simulink model "forceControl"  (R2024b)
settings: Solver=VariableStepAuto  StartTime=0.0  StopTime=10
values from neighbouring files (symbols this model uses):
  robotStructure = block.DialogPrm(1).Data    [activeCompliance.m]    (also in robot.mat = )
undefined symbols (not defined in the file or in its folder): X, Y, Z
libraries: sm_lib x141, nesl_utility x12, matrix_library x3
(part 1 of 3)
settings Model: PacingRate=10000  Creator=luca  LastModifiedBy=luca
settings DebuggingCC: AlgebraicLoopMsg=none

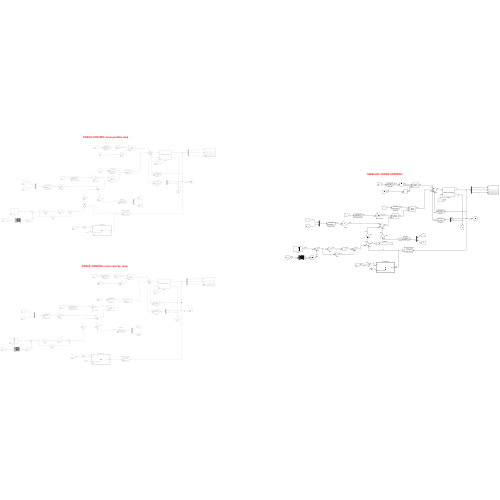
[thumbnail: Simulink's stored preview of the top-level diagram]
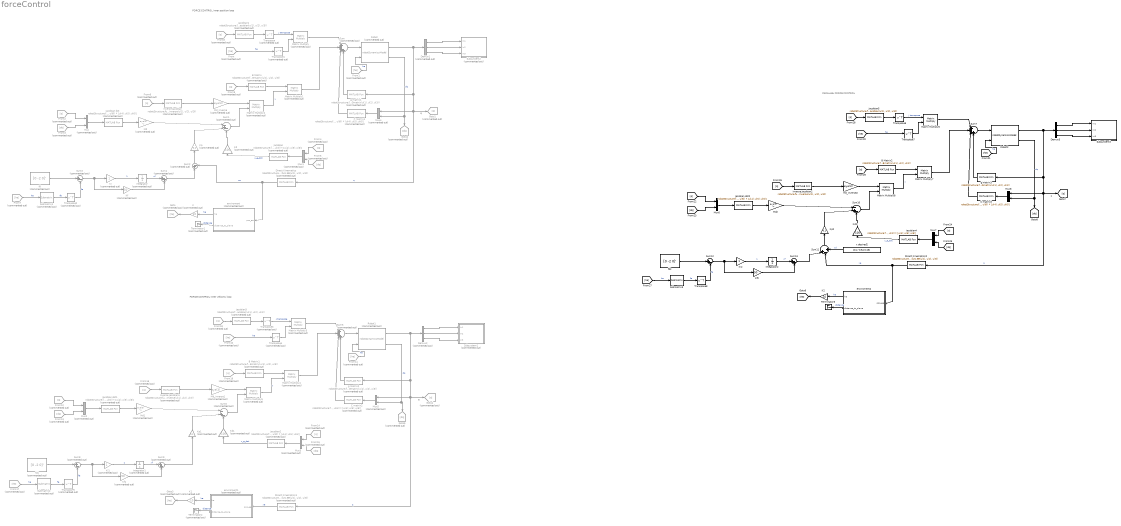
== system forceControl ==
  note: q
  note: FORCE CONTROL inner position loop
  note: q
  note: FORCE CONTROL inner velocity loop
  note: q
  note: PARALLEL FORCE CONTROL
  B Matrix : MATLABFcn  Commented=on  MATLABFcn=robotStructure.func.Bmatrix(u(1), u(2), u(3))  Output1D=off
  B Matrix1 : MATLABFcn  Commented=on  MATLABFcn=robotStructure.func.Bmatrix(u(1), u(2), u(3))  Output1D=off
  B Matrix2 : MATLABFcn  MATLABFcn=robotStructure.func.Bmatrix(u(1), u(2), u(3))  Output1D=off
  C matrix1 : MATLABFcn  Commented=on  MATLABFcn=robotStructure.func.Cmatrix(u(1), u(2), u(3), u(4), u(5), u(6)) * [u(4); u(5); u(6)]  OutputSignalType=real  Output1D=off
  C matrix2 : MATLABFcn  Commented=on  MATLABFcn=robotStructure.func.Cmatrix(u(1), u(2), u(3), u(4), u(5), u(6)) * [u(4); u(5); u(6)]  OutputSignalType=real  Output1D=off
  C matrix3 : MATLABFcn  MATLABFcn=robotStructure.func.Cmatrix(u(1), u(2), u(3), u(4), u(5), u(6)) * [u(4); u(5); u(6)]  OutputSignalType=real  Output1D=off
  Demux1 : Demux  Commented=on  Outputs=3
  Demux2 : Demux  Commented=on  Outputs=3
  Demux3 : Demux  Outputs=3
  Direct Kinematics : MATLABFcn  Commented=on  MATLABFcn=robotStructure.func.EE(u(1), u(2), u(3))  Output1D=off
  Direct Kinematics1 : MATLABFcn  Commented=on  MATLABFcn=robotStructure.func.EE(u(1), u(2), u(3))  Output1D=off
  Direct Kinematics2 : MATLABFcn  MATLABFcn=robotStructure.func.EE(u(1), u(2), u(3))  Output1D=off
  From{,1,7,10..11,17} (6 alike) : From  Commented=on  GotoTag=he
  From{2,4,6,8..9,12,14,16,18..19} (10 alike) : From  Commented=on  GotoTag=q
  From{3,5,13,15} (4 alike) : From  Commented=on  GotoTag=dq
  Goto : Goto  Commented=on  GotoTag=he
  Goto1 : Goto  Commented=on  GotoTag=q
  Goto2 : Goto  Commented=on  GotoTag=dq
  Goto3 : Goto  Commented=on  GotoTag=he
  Goto4 : Goto  Commented=on  GotoTag=q
  Goto5 : Goto  Commented=on  GotoTag=dq
  Integrator : Integrator  Commented=on
  Integrator1 : Integrator  Commented=on
  Integrator2 : Integrator
  K : Gain  Commented=on  Gain=10
  K1 : Gain  Commented=on  Gain=10
  K2 : Gain  Gain=10
  Kd : Gain  Commented=on  Gain=100
  Kd1 : Gain  Commented=on  Gain=100
  Kd2 : Gain  Gain=100
  Kf : Gain  Commented=on  Gain=50
  Kf1 : Gain  Commented=on  Gain=50
  Kf2 : Gain  Gain=50
  Ki : Gain  Commented=on
  Ki1 : Gain  Commented=on
  Ki2 : Gain
  Kp : Gain  Commented=on  Gain=0.1
  Kp1 : Gain  Commented=on  Gain=0.1
  Kp2 : Gain  Gain=0.1
  Matrix Multiply{,1..5} (6 alike) : Product  Commented=on  Multiplication=Matrix(*)
  Matrix Multiply6 : Product  Multiplication=Matrix(*)
  Matrix Multiply7 : Product  Multiplication=Matrix(*)
  Matrix Multiply8 : Product  Multiplication=Matrix(*)
  Md : Gain  Commented=on  Gain=eye(3)  Multiplication=Matrix(K*u)
  Md1 : Gain  Commented=on  Gain=eye(3)  Multiplication=Matrix(K*u)
  Md2 : Gain  Gain=eye(3)  Multiplication=Matrix(K*u)
  Md_inverse : Gain  Commented=on  Gain=eye(3)
  Md_inverse1 : Gain  Commented=on  Gain=eye(3)
  Md_inverse2 : Gain  Gain=eye(3)
  Mux{,1..5} (6 alike) : Mux  Commented=on  Inputs=2
  Mux6 : Mux  Inputs=2
  Mux7 : Mux  Inputs=2
  Mux8 : Mux  Inputs=2
  Robot : M-S-Function  Commented=on  FunctionName=robotDynamicsModel  Parameters=robotStructure, [0 -0.05 0], [0 0 0]
  Robot1 : M-S-Function  Commented=on  FunctionName=robotDynamicsModel  Parameters=robotStructure, [0 -0.05 0], [0 0 0]
  Robot2 : M-S-Function  FunctionName=robotDynamicsModel  Parameters=robotStructure, [0 -0.2 0], [0 0 0]
  Submatrix1 : matrix_library/Submatrix  Commented=on  RowSpan=All rows  RowStartMode=Index  RowStartIndex=1  RowEndMode=Index  RowEndIndex=1  ColSpan=Range of columns  ColStartMode=Index  ColStartIndex=1  ColEndMode=Index  ColEndIndex=3
  Submatrix2 : matrix_library/Submatrix  Commented=on  RowSpan=All rows  RowStartMode=Index  RowStartIndex=1  RowEndMode=Index  RowEndIndex=1  ColSpan=Range of columns  ColStartMode=Index  ColStartIndex=1  ColEndMode=Index  ColEndIndex=3
  Submatrix3 : matrix_library/Submatrix  RowSpan=All rows  RowStartMode=Index  RowStartIndex=1  RowEndMode=Index  RowEndIndex=1  ColSpan=Range of columns  ColStartMode=Index  ColStartIndex=1  ColEndMode=Index  ColEndIndex=3
  Subsystem1 : Subsystem  Commented=on
  Subsystem2 : Subsystem  Commented=on
  Subsystem3 : Subsystem
  Sum : Sum  Commented=on  Inputs=|++++
  Sum1 : Sum  Commented=on  Inputs=|-+-
  Sum10 : Sum  Inputs=|-+-
  Sum11 : Sum  Inputs=|+|-|+
  Sum12 : Sum  Inputs=|+-
  Sum13 : Sum  Inputs=|++
  Sum2 : Sum  Commented=on  Inputs=|+-
  Sum3 : Sum  Commented=on  Inputs=|+-
  Sum4 : Sum  Commented=on  Inputs=|++
  Sum5 : Sum  Commented=on  Inputs=|++++
  Sum6 : Sum  Commented=on  Inputs=|-+-
  Sum7 : Sum  Inputs=|++++
  Sum8 : Sum  Commented=on  Inputs=|+-
  Sum9 : Sum  Commented=on  Inputs=|++
  Terminator1 : Terminator  Commented=on
  Terminator2 : Terminator  Commented=on
  Terminator3 : Terminator
  Transpose{,1..5} (6 alike) : Math  Commented=on  Operator=transpose
  Transpose6 : Math  Operator=transpose
  Transpose7 : Math  Operator=transpose
  Transpose8 : Math  Operator=transpose
  enviroment : MATLAB Function  Commented=on  TreatAsAtomicUnit=on
  enviroment1 : MATLAB Function  Commented=on  TreatAsAtomicUnit=on
  enviroment2 : MATLAB Function  TreatAsAtomicUnit=on
  fd : Constant  Commented=on  Value=[0 -2 0]'  VectorParams1D=off
  fd1 : Constant  Commented=on  Value=[0 -2 0]'  VectorParams1D=off
  fd2 : Constant  Value=[0 -2 0]'  VectorParams1D=off
  g matrix1 : MATLABFcn  Commented=on  MATLABFcn=robotStructure.func.Gmatrix(u(1), u(2), u(3))  OutputSignalType=real  Output1D=off
  g matrix2 : MATLABFcn  Commented=on  MATLABFcn=robotStructure.func.Gmatrix(u(1), u(2), u(3))  OutputSignalType=real  Output1D=off
  g matrix3 : MATLABFcn  MATLABFcn=robotStructure.func.Gmatrix(u(1), u(2), u(3))  OutputSignalType=real  Output1D=off
  inverse Jacobian : MATLABFcn  Commented=on  MATLABFcn=robotStructure.func.AnalitycalJacobianInverse(u(1), u(2), u(3))  Output1D=off
  inverse Jacobian1 : MATLABFcn  Commented=on  MATLABFcn=robotStructure.func.AnalitycalJacobianInverse(u(1), u(2), u(3))  Output1D=off
  inverse Jacobian2 : MATLABFcn  MATLABFcn=robotStructure.func.AnalitycalJacobianInverse(u(1), u(2), u(3))  Output1D=off
  jacobian : MATLABFcn  Commented=on  MATLABFcn=robotStructure.func.AnalitycalJacobian(u(1), u(2), u(3)) * [u(4); u(5); u(6)]  Output1D=off
  jacobian dot : MATLABFcn  Commented=on  MATLABFcn=robotStructure.func.AnalitycalJacobianDot(u(1), u(2), u(3), u(4), u(5), u(6)) * [u(4); u(5); u(6)]  Output1D=off
  jacobian dot1 : MATLABFcn  Commented=on  MATLABFcn=robotStructure.func.AnalitycalJacobianDot(u(1), u(2), u(3), u(4), u(5), u(6)) * [u(4); u(5); u(6)]  Output1D=off
  jacobian dot2 : MATLABFcn  MATLABFcn=robotStructure.func.AnalitycalJacobianDot(u(1), u(2), u(3), u(4), u(5), u(6)) * [u(4); u(5); u(6)]  Output1D=off
  jacobian1 : MATLABFcn  Commented=on  MATLABFcn=robotStructure.func.GeometricJacobian(u(1), u(2), u(3))  Output1D=off
  jacobian2 : MATLABFcn  Commented=on  MATLABFcn=robotStructure.func.AnalitycalJacobian(u(1), u(2), u(3)) * [u(4); u(5); u(6)]  Output1D=off
  jacobian3 : MATLABFcn  Commented=on  MATLABFcn=robotStructure.func.GeometricJacobian(u(1), u(2), u(3))  Output1D=off
  jacobian4 : MATLABFcn  MATLABFcn=robotStructure.func.AnalitycalJacobian(u(1), u(2), u(3)) * [u(4); u(5); u(6)]  Output1D=off
  jacobian5 : MATLABFcn  MATLABFcn=robotStructure.func.GeometricJacobian(u(1), u(2), u(3))  Output1D=off
  x desired2 : Constant  Value=[0.4 -0.54 0.15]
  wires:
  enviroment/2(distance_to_plane) -> Terminator1/1  "distance"
  Demux1/2 -> Subsystem2/2(In2)
  Robot/1 -> g matrix1/1, Goto1/1, Mux4/1, Direct Kinematics/1, Demux1/1  "q"
  Demux1/1 -> Subsystem2/1(In1)
  Demux1/3 -> Subsystem2/3(In3)
  Sum/1 -> Robot/1
  Robot/2 -> Mux4/2, Goto2/1  "dq"
  Mux4/1 -> C matrix1/1
  enviroment/1(he) -> K/1  "he"
  g matrix1/1 -> Sum/4
  C matrix1/1 -> Sum/3
  From1/1 -> Robot/2  "he"
  Direct Kinematics/1 -> Sum2/2, enviroment/1(pos_ee)  "xe"
  B Matrix/1 -> Matrix Multiply1/1
  Matrix Multiply2/1 -> Matrix Multiply1/2  "y"
  inverse Jacobian/1 -> Md_inverse/1
  Md_inverse/1 -> Matrix Multiply2/1
  Sum1/1 -> Matrix Multiply2/2
  Kd/1 -> Sum1/3
  jacobian/1 -> Kd/1  "x_e_dot"
  Kp/1 -> Sum1/2
  Sum2/1 -> Kp/1
  jacobian dot/1 -> Md/1
  Md/1 -> Sum1/1
  From2/1 -> Mux/1
  Mux/1 -> jacobian dot/1
  From3/1 -> Mux/2
  From/1 -> Transpose1/1  "he"
  From5/1 -> Mux1/2
  From4/1 -> Mux1/1
  Mux1/1 -> jacobian/1
  From6/1 -> inverse Jacobian/1
  From9/1 -> B Matrix/1
  Transpose2/1 -> Sum3/2  "fe"
  Submatrix1/1 -> Transpose2/1  "fe"
  From7/1 -> Submatrix1/1  "he"
  fd/1 -> Sum3/1
  Sum3/1 -> Kf/1, Ki/1
  Ki/1 -> Integrator/1  "1"
  Integrator/1 -> Sum4/1  "xf"
  Sum4/1 -> Sum2/1
  K/1 -> Goto/1
  Matrix Multiply1/1 -> Sum/2
  Matrix Multiply/1 -> Sum/1
  From8/1 -> jacobian1/1
  jacobian1/1 -> Transpose/1
  Transpose/1 -> Matrix Multiply/1  "J transpose"
  Transpose1/1 -> Matrix Multiply/2
  Kf/1 -> Sum4/2
  Sum8/1 -> Kf1/1, Ki1/1
  Kf1/1 -> Sum9/2
  From17/1 -> Submatrix2/1  "he"
  Md1/1 -> Sum6/1
  inverse Jacobian1/1 -> Md_inverse1/1
  g matrix2/1 -> Sum5/4
  Ki1/1 -> Integrator1/1  "1"
  Mux5/1 -> C matrix2/1
  C matrix2/1 -> Sum5/3
  Robot1/1 -> g matrix2/1, Goto4/1, Mux5/1, Direct Kinematics1/1, Demux2/1  "q"
  enviroment1/2(distance_to_plane) -> Terminator2/1  "distance"
  From19/1 -> B Matrix1/1
  From16/1 -> inverse Jacobian1/1
  From13/1 -> Mux2/2
  Direct Kinematics1/1 -> enviroment1/1(pos_ee)  "xe"
  Sum6/1 -> Matrix Multiply5/2
  Matrix Multiply3/1 -> Sum5/1
  Sum5/1 -> Robot1/1
  B Matrix1/1 -> Matrix Multiply4/1
  From11/1 -> Robot1/2  "he"
  Transpose4/1 -> Matrix Multiply3/2
  K1/1 -> Goto3/1
  Mux3/1 -> jacobian2/1
  Transpose5/1 -> Sum8/2  "fe"
  enviroment1/1(he) -> K1/1  "he"
  jacobian3/1 -> Transpose3/1
  From15/1 -> Mux3/2
  Demux2/2 -> Subsystem1/2(In2)
  Integrator1/1 -> Sum9/1  "xf"
  Matrix Multiply5/1 -> Matrix Multiply4/2  "y"
  Kp1/1 -> Sum6/2
  From14/1 -> Mux3/1
  Matrix Multiply4/1 -> Sum5/2
  From10/1 -> Transpose4/1  "he"
  From12/1 -> Mux2/1
  From18/1 -> jacobian3/1
  Md_inverse1/1 -> Matrix Multiply5/1
  Mux2/1 -> jacobian dot1/1
  Robot1/2 -> Mux5/2, Goto5/1  "dq"
  Transpose3/1 -> Matrix Multiply3/1  "J transpose"
  Submatrix2/1 -> Transpose5/1  "fe"
  jacobian dot1/1 -> Md1/1
  jacobian2/1 -> Kd1/1  "x_e_dot"
  Demux2/3 -> Subsystem1/3(In3)
  Kd1/1 -> Sum6/3
  fd1/1 -> Sum8/1
  Demux2/1 -> Subsystem1/1(In1)
  Sum9/1 -> Kp1/1
  Sum12/1 -> Kf2/1, Ki2/1
  Kf2/1 -> Sum13/2
  [he] -> Submatrix3/1  "he"
  Md2/1 -> Sum10/1
  inverse Jacobian2/1 -> Md_inverse2/1
  g matrix3/1 -> Sum7/4
  Ki2/1 -> Integrator2/1  "1"
  Mux8/1 -> C matrix3/1
  C matrix3/1 -> Sum7/3
  Robot2/1 -> g matrix3/1, [q], Mux8/1, Direct Kinematics2/1, Demux3/1  "q"
  enviroment2/2(distance_to_plane) -> Terminator3/1  "distance"
  [q] -> B Matrix2/1
  [q] -> inverse Jacobian2/1
  [dq] -> Mux6/2
  Direct Kinematics2/1 -> Sum11/2, enviroment2/1(pos_ee)  "xe"
  Sum10/1 -> Matrix Multiply8/2
  Matrix Multiply6/1 -> Sum7/1
  Sum7/1 -> Robot2/1
  B Matrix2/1 -> Matrix Multiply7/1
  [he] -> Robot2/2  "he"
  Transpose7/1 -> Matrix Multiply6/2
  K2/1 -> [he]
  Mux7/1 -> jacobian4/1
  Transpose8/1 -> Sum12/2  "fe"
  enviroment2/1(he) -> K2/1  "he"
  jacobian5/1 -> Transpose6/1
  [dq] -> Mux7/2
  Demux3/2 -> Subsystem3/2(In2)
  Integrator2/1 -> Sum13/1  "xf"
  Matrix Multiply8/1 -> Matrix Multiply7/2  "y"
  Kp2/1 -> Sum10/2
  [q] -> Mux7/1
  Matrix Multiply7/1 -> Sum7/2
  [he] -> Transpose7/1  "he"
  [q] -> Mux6/1
  Sum13/1 -> Sum11/1
  [q] -> jacobian5/1
  Md_inverse2/1 -> Matrix Multiply8/1
  Mux6/1 -> jacobian dot2/1
  Robot2/2 -> Mux8/2, [dq]  "dq"
  Transpose6/1 -> Matrix Multiply6/1  "J transpose"
  Submatrix3/1 -> Transpose8/1  "fe"
  jacobian dot2/1 -> Md2/1
  jacobian4/1 -> Kd2/1  "x_e_dot"
  Demux3/3 -> Subsystem3/3(In3)
  Kd2/1 -> Sum10/3
  fd2/1 -> Sum12/1
  Demux3/1 -> Subsystem3/1(In1)
  Sum11/1 -> Kp2/1
  x desired2/1 -> Sum11/3  "xd"

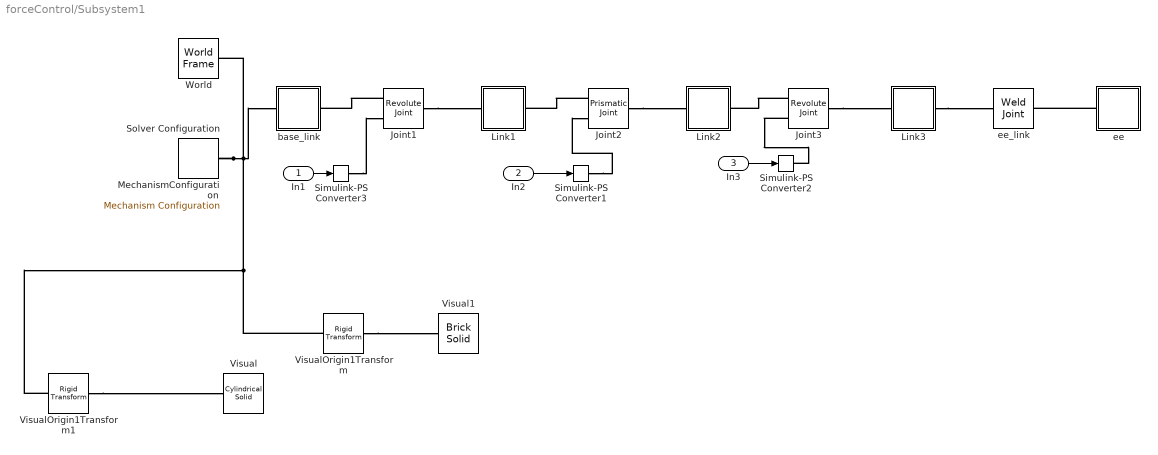
== system forceControl/Subsystem1 ==
  In1 : Inport
  In2 : Inport  Port=2
  In3 : Inport  Port=3
  Joint1 : sm_lib/Joints/Revolute Joint  JointMode=Normal  CompositeWrenchDir=FollowerOnBase  CompositeWrenchFrame=BaseFrame  SenseConstraintForce=off  SenseConstraintTorque=off  SenseTotalForce=off  SenseTotalTorque=off  PositionTargetSpecify=off  PositionTargetPriority=High  PositionTargetValue=0  PositionTargetValueUnits=deg  VelocityTargetSpecify=off  VelocityTargetPriority=High  VelocityTargetValue=0  VelocityTargetValueUnits=deg/s  EquilibriumPosition=0  EquilibriumPositionUnits=deg  SpringStiffness=0  SpringStiffnessUnits=N*m/deg  DampingCoefficient=0  DampingCoefficientUnits=kg*m^2/(rad*s)  LowerLimitSpecify=on  LowerLimitBound=-3.14  LowerLimitBoundUnits=rad  LowerLimitStiffness=1e4  LowerLimitStiffnessUnits=N*m/deg  LowerLimitDamping=10  LowerLimitDampingUnits=N*m/(deg/s)  LowerLimitTransitionRegionWidth=0.1  LowerLimitTransitionRegionWidthUnits=deg  UpperLimitSpecify=on  UpperLimitBound=3.14  UpperLimitBoundUnits=rad  UpperLimitStiffness=1e4  UpperLimitStiffnessUnits=N*m/deg  UpperLimitDamping=10  UpperLimitDampingUnits=N*m/(deg/s)  UpperLimitTransitionRegionWidth=0.1  UpperLimitTransitionRegionWidthUnits=deg  TorqueActuationMode=ComputedTorque  MotionActuationMode=InputMotion  SensePosition=off  SenseVelocity=off  SenseAcceleration=off  SenseTorqueForce=off  SenseLowerLimitTorqueForce=off  SenseUpperLimitTorqueForce=off
  Joint2 : sm_lib/Joints/Prismatic Joint  JointMode=Normal  CompositeWrenchDir=FollowerOnBase  CompositeWrenchFrame=BaseFrame  SenseConstraintForce=off  SenseConstraintTorque=off  SenseTotalForce=off  SenseTotalTorque=off  PositionTargetSpecify=off  PositionTargetPriority=High  PositionTargetValue=0  PositionTargetValueUnits=m  VelocityTargetSpecify=off  VelocityTargetPriority=High  VelocityTargetValue=0  VelocityTargetValueUnits=m/s  EquilibriumPosition=0  EquilibriumPositionUnits=m  SpringStiffness=0  SpringStiffnessUnits=N/m  DampingCoefficient=0  DampingCoefficientUnits=kg/s  LowerLimitSpecify=on  LowerLimitBound=-0.3  LowerLimitBoundUnits=m  LowerLimitStiffness=1e6  LowerLimitStiffnessUnits=N/m  LowerLimitDamping=1e3  LowerLimitDampingUnits=N/(m/s)  LowerLimitTransitionRegionWidth=1e-4  LowerLimitTransitionRegionWidthUnits=m  UpperLimitSpecify=on  UpperLimitBound=0  UpperLimitBoundUnits=m  UpperLimitStiffness=1e6  UpperLimitStiffnessUnits=N/m  UpperLimitDamping=1e3  UpperLimitDampingUnits=N/(m/s)  UpperLimitTransitionRegionWidth=1e-4  UpperLimitTransitionRegionWidthUnits=m  TorqueActuationMode=ComputedTorque  MotionActuationMode=InputMotion  SensePosition=off  SenseVelocity=off  SenseAcceleration=off  SenseTorqueForce=off  SenseLowerLimitTorqueForce=off  SenseUpperLimitTorqueForce=off
  Joint3 : sm_lib/Joints/Revolute Joint  JointMode=Normal  CompositeWrenchDir=FollowerOnBase  CompositeWrenchFrame=BaseFrame  SenseConstraintForce=off  SenseConstraintTorque=off  SenseTotalForce=off  SenseTotalTorque=off  PositionTargetSpecify=off  PositionTargetPriority=High  PositionTargetValue=0  PositionTargetValueUnits=deg  VelocityTargetSpecify=off  VelocityTargetPriority=High  VelocityTargetValue=0  VelocityTargetValueUnits=deg/s  EquilibriumPosition=0  EquilibriumPositionUnits=deg  SpringStiffness=0  SpringStiffnessUnits=N*m/deg  DampingCoefficient=0  DampingCoefficientUnits=kg*m^2/(rad*s)  LowerLimitSpecify=on  LowerLimitBound=-3.14  LowerLimitBoundUnits=rad  LowerLimitStiffness=1e4  LowerLimitStiffnessUnits=N*m/deg  LowerLimitDamping=10  LowerLimitDampingUnits=N*m/(deg/s)  LowerLimitTransitionRegionWidth=0.1  LowerLimitTransitionRegionWidthUnits=deg  UpperLimitSpecify=on  UpperLimitBound=3.14  UpperLimitBoundUnits=rad  UpperLimitStiffness=1e4  UpperLimitStiffnessUnits=N*m/deg  UpperLimitDamping=10  UpperLimitDampingUnits=N*m/(deg/s)  UpperLimitTransitionRegionWidth=0.1  UpperLimitTransitionRegionWidthUnits=deg  TorqueActuationMode=ComputedTorque  MotionActuationMode=InputMotion  SensePosition=off  SenseVelocity=off  SenseAcceleration=off  SenseTorqueForce=off  SenseLowerLimitTorqueForce=off  SenseUpperLimitTorqueForce=off
  Link1 : Subsystem
  Link2 : Subsystem
  Link3 : Subsystem
  MechanismConfiguration : sm_lib/Utilities/Mechanism Configuration  UniformGravity=Constant  GravityVector=[0 0 -9.80665]  GravityVectorUnits=m/s^2  LinearizationDelta=0.001  JointModeTransitionNonlinearIterations=2
  Simulink-PS Converter1 : nesl_utility/Simulink-PS Converter  PhysicalDomain=network_engine_domain  SubClassName=ps_input  LeftPortType=input  RightPortType=output  PseudoPeriodic=off  Frequencies=[]  NoiseDistribution=none  NoiseParameters=[]  Unit=1  AffineConversion=off  FilteringAndDerivatives=filter  SimscapeFilterOrder=2  InputFilterTimeConstant=0.001  UdotUserProvided=0
  Simulink-PS Converter2 : nesl_utility/Simulink-PS Converter  PhysicalDomain=network_engine_domain  SubClassName=ps_input  LeftPortType=input  RightPortType=output  PseudoPeriodic=off  Frequencies=[]  NoiseDistribution=none  NoiseParameters=[]  Unit=1  AffineConversion=off  FilteringAndDerivatives=filter  SimscapeFilterOrder=2  InputFilterTimeConstant=0.001  UdotUserProvided=0
  Simulink-PS Converter3 : nesl_utility/Simulink-PS Converter  PhysicalDomain=network_engine_domain  SubClassName=ps_input  LeftPortType=input  RightPortType=output  PseudoPeriodic=off  Frequencies=[]  NoiseDistribution=none  NoiseParameters=[]  Unit=1  AffineConversion=off  FilteringAndDerivatives=filter  SimscapeFilterOrder=2  InputFilterTimeConstant=0.001  UdotUserProvided=0
  Solver Configuration : nesl_utility/Solver Configuration  PhysicalDomain=network_engine_domain  SubClassName=solver  LeftPortType=input  RightPortType=generic  Tones=[]  Harmonics=[]  SimulateNoise=off  Profile=off  UseLocalSampling=off  EnableSwitchedLinearOptims=on  FrequencyDomain=off  UseCCode=off  RelTol=0.001  AbsTol=0.001  MinStep=1e-09  ToWorkspace=off  RevertToSquareIcSolve=off  NumHomotopyIterations=100  PhasorMode=off  PhasorModeNumHarmonics=1  ConsistencySolver=NEWTON_XTOL_AFTER_FTOL  IndexReductionMethod=DerivativeReplacement  DoDC=off  ResidualTolerance=1e-09  ConsistencyTolSource=GLOBAL  ConsistencyAbsTol=0.001  ConsistencyRelTol=0.001  ConsistencyTolFactor=0.001  UseLocalSolver=off  LocalSolverChoice=NE_BACKWARD_EULER_ADVANCER  ResolveIndetEquations=on  FunctionEvalNumThread=1  LocalSolverSampleTime=0.001  DoFixedCost=off  MaxNonlinIter=3  MaxModeIter=2  ComputeImpulses=off  ImpulseIterations=2  LinearAlgebra=auto  LinearAlgebraNumThread=0  EquationFormulation=NE_TIME_EF  DelaysMemoryBudget=1024  AutomaticFiltering=on  FilteringTimeConstant=0.001  PartitionStorageMethod=AS_NEEDED  PartitionMemoryBudget=1024  PartitionMethod=ROBUST  MultibodyUseLocalSolver=off  MultibodyLocalSolverChoice=ODE1  MultibodyLocalSolverSampleTime=0.001
  Visual : sm_lib/Body Elements/Cylindrical Solid  CylinderRadius=0.02  CylinderRadiusUnits=m  CylinderLength=0.01  CylinderLengthUnits=m  ExportEntireGeometry=off  InertiaType=Custom  BasedOnType=Density  Density=1000  DensityUnits=kg/m^3  Mass=0  MassUnits=kg  CenterOfMass=[0, 0, 0]  CenterOfMassUnits=m  MomentsOfInertia=[0, 0, 0]  MomentsOfInertiaUnits=kg*m^2  ProductsOfInertia=[0, 0, 0]  ProductsOfInertiaUnits=kg*m^2  GraphicType=FromGeometry  MarkerShape=Sphere  MarkerSize=10  GraphicVisPropType=SimpleVisualProperties  GraphicDiffuseColor=[1, 1, 0]  GraphicOpacity=1  GraphicSpecularColor=[0.5 0.5 0.5 1.0]  GraphicAmbientColor=[0.15 0.15 0.15 1.0]  GraphicEmissiveColor=[0.0 0.0 0.0 1.0]  GraphicShininess=75  DoExposeReferenceFrame=on  SerializedFrames=<Frames/>
  Visual1 : sm_lib/Body Elements/Brick Solid  BrickDimensions=[0.4, 0.4, 0.1]  BrickDimensionsUnits=m  ExportEntireGeometry=off  InertiaType=Custom  BasedOnType=Density  Density=1000  DensityUnits=kg/m^3  Mass=0  MassUnits=kg  CenterOfMass=[0, 0, 0]  CenterOfMassUnits=m  MomentsOfInertia=[0, 0, 0]  MomentsOfInertiaUnits=kg*m^2  ProductsOfInertia=[0, 0, 0]  ProductsOfInertiaUnits=kg*m^2  GraphicType=FromGeometry  MarkerShape=Sphere  MarkerSize=10  GraphicVisPropType=SimpleVisualProperties  GraphicDiffuseColor=[1 0.4118 0.1608]  GraphicOpacity=0.6  GraphicSpecularColor=[0.5 0.5 0.5 1.0]  GraphicAmbientColor=[0.15 0.15 0.15 1.0]  GraphicEmissiveColor=[0.0 0.0 0.0 1.0]  GraphicShininess=75  DoExposeReferenceFrame=on  SerializedFrames=<Frames/>
  VisualOrigin1Transform : sm_lib/Frames and Transforms/Rigid Transform  RotationMethod=RotationSequence  FollAlignAxisA=+X  BaseAlignAxisA=+Y  FollAlignAxisB=+Y  BaseAlignAxisB=+Z  RotationStandardAxis=+Z  RotationAngle=0  RotationAngleUnits=deg  RotationArbitraryAxis=[0 0 1]  RotationSequenceAxes=BaseAxes  RotationSequence=XYZ  RotationSequenceAngles=[pi/2, 0, 0]  RotationSequenceAnglesUnits=rad  RotationMatrix=[1 0 0;0 1 0;0 0 1]  Quaternion=[1 0 0 0]  TranslationMethod=Cartesian  TranslationCartesianOffset=[0.4, -0.45, 0.2]  TranslationCartesianOffsetUnits=m  TranslationStandardAxis=+Z  TranslationStandardOffset=0  TranslationStandardOffsetUnits=m  TranslationROffset=0  TranslationROffsetUnits=m  TranslationThetaOffset=0  TranslationThetaOffsetUnits=deg  TranslationZOffset=0  TranslationZOffsetUnits=m
  VisualOrigin1Transform1 : sm_lib/Frames and Transforms/Rigid Transform  RotationMethod=RotationSequence  FollAlignAxisA=+X  BaseAlignAxisA=+Y  FollAlignAxisB=+Y  BaseAlignAxisB=+Z  RotationStandardAxis=+Z  RotationAngle=0  RotationAngleUnits=deg  RotationArbitraryAxis=[0 0 1]  RotationSequenceAxes=BaseAxes  RotationSequence=XYZ  RotationSequenceAngles=[0, 0, 0]  RotationSequenceAnglesUnits=rad  RotationMatrix=[1 0 0;0 1 0;0 0 1]  Quaternion=[1 0 0 0]  TranslationMethod=Cartesian  TranslationCartesianOffset=[0.4 -0.54 0.15]  TranslationCartesianOffsetUnits=m  TranslationStandardAxis=+Z  TranslationStandardOffset=0  TranslationStandardOffsetUnits=m  TranslationROffset=0  TranslationROffsetUnits=m  TranslationThetaOffset=0  TranslationThetaOffsetUnits=deg  TranslationZOffset=0  TranslationZOffsetUnits=m
  World : sm_lib/Frames and Transforms/World Frame
  base_link : Subsystem
  ee : Subsystem
  ee_link : sm_lib/Joints/Weld Joint  JointMode=Normal  CompositeWrenchDir=FollowerOnBase  CompositeWrenchFrame=BaseFrame  SenseConstraintForce=off  SenseConstraintTorque=off  SenseTotalForce=off  SenseTotalTorque=off
  wires:
  In3/1 -> Simulink-PS Converter2/1
  In1/1 -> Simulink-PS Converter3/1
  In2/1 -> Simulink-PS Converter1/1
  connections:
  Simulink-PS Converter3/RConn1 -- Joint1/LConn2
  Simulink-PS Converter1/RConn1 -- Joint2/LConn2
  Joint3/LConn2 -- Simulink-PS Converter2/RConn1
  World/RConn1 -- VisualOrigin1Transform1/LConn1 -- VisualOrigin1Transform/LConn1 -- base_link/LConn1 -- MechanismConfiguration/RConn1 -- Solver Configuration/RConn1
  Joint2/RConn1 -- Link2/LConn1
  Joint2/LConn1 -- Link1/RConn1
  Joint3/LConn1 -- Link2/RConn1
  Link3/RConn1 -- ee_link/LConn1
  ee/LConn1 -- ee_link/RConn1
  Joint1/RConn1 -- Link1/LConn1
  Joint3/RConn1 -- Link3/LConn1
  Joint1/LConn1 -- base_link/RConn1
  VisualOrigin1Transform/RConn1 -- Visual1/RConn1
  VisualOrigin1Transform1/RConn1 -- Visual/RConn1

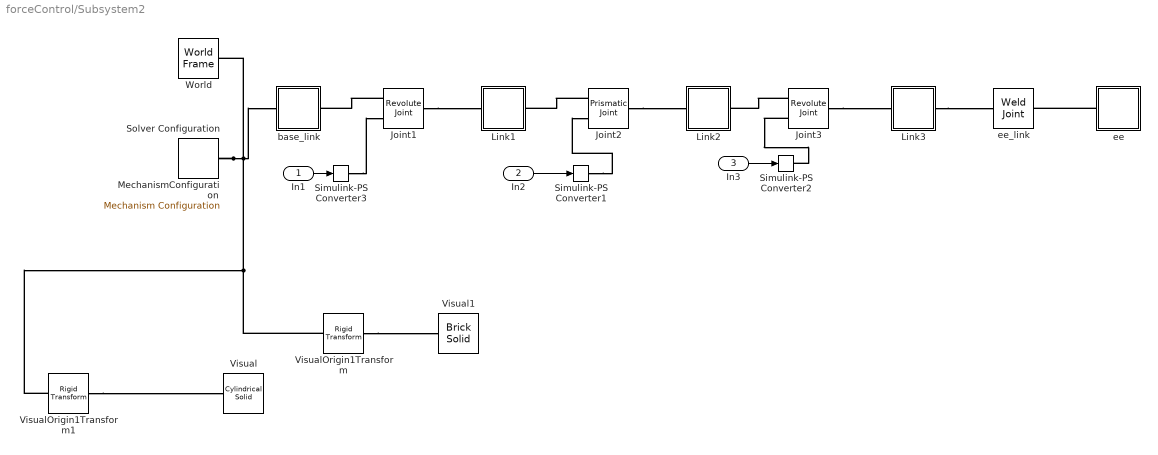
== system forceControl/Subsystem2 ==
  In1 : Inport
  In2 : Inport  Port=2
  In3 : Inport  Port=3
  Joint1 : sm_lib/Joints/Revolute Joint  JointMode=Normal  CompositeWrenchDir=FollowerOnBase  CompositeWrenchFrame=BaseFrame  SenseConstraintForce=off  SenseConstraintTorque=off  SenseTotalForce=off  SenseTotalTorque=off  PositionTargetSpecify=off  PositionTargetPriority=High  PositionTargetValue=0  PositionTargetValueUnits=deg  VelocityTargetSpecify=off  VelocityTargetPriority=High  VelocityTargetValue=0  VelocityTargetValueUnits=deg/s  EquilibriumPosition=0  EquilibriumPositionUnits=deg  SpringStiffness=0  SpringStiffnessUnits=N*m/deg  DampingCoefficient=0  DampingCoefficientUnits=kg*m^2/(rad*s)  LowerLimitSpecify=on  LowerLimitBound=-3.14  LowerLimitBoundUnits=rad  LowerLimitStiffness=1e4  LowerLimitStiffnessUnits=N*m/deg  LowerLimitDamping=10  LowerLimitDampingUnits=N*m/(deg/s)  LowerLimitTransitionRegionWidth=0.1  LowerLimitTransitionRegionWidthUnits=deg  UpperLimitSpecify=on  UpperLimitBound=3.14  UpperLimitBoundUnits=rad  UpperLimitStiffness=1e4  UpperLimitStiffnessUnits=N*m/deg  UpperLimitDamping=10  UpperLimitDampingUnits=N*m/(deg/s)  UpperLimitTransitionRegionWidth=0.1  UpperLimitTransitionRegionWidthUnits=deg  TorqueActuationMode=ComputedTorque  MotionActuationMode=InputMotion  SensePosition=off  SenseVelocity=off  SenseAcceleration=off  SenseTorqueForce=off  SenseLowerLimitTorqueForce=off  SenseUpperLimitTorqueForce=off
  Joint2 : sm_lib/Joints/Prismatic Joint  JointMode=Normal  CompositeWrenchDir=FollowerOnBase  CompositeWrenchFrame=BaseFrame  SenseConstraintForce=off  SenseConstraintTorque=off  SenseTotalForce=off  SenseTotalTorque=off  PositionTargetSpecify=off  PositionTargetPriority=High  PositionTargetValue=0  PositionTargetValueUnits=m  VelocityTargetSpecify=off  VelocityTargetPriority=High  VelocityTargetValue=0  VelocityTargetValueUnits=m/s  EquilibriumPosition=0  EquilibriumPositionUnits=m  SpringStiffness=0  SpringStiffnessUnits=N/m  DampingCoefficient=0  DampingCoefficientUnits=kg/s  LowerLimitSpecify=on  LowerLimitBound=-0.3  LowerLimitBoundUnits=m  LowerLimitStiffness=1e6  LowerLimitStiffnessUnits=N/m  LowerLimitDamping=1e3  LowerLimitDampingUnits=N/(m/s)  LowerLimitTransitionRegionWidth=1e-4  LowerLimitTransitionRegionWidthUnits=m  UpperLimitSpecify=on  UpperLimitBound=0  UpperLimitBoundUnits=m  UpperLimitStiffness=1e6  UpperLimitStiffnessUnits=N/m  UpperLimitDamping=1e3  UpperLimitDampingUnits=N/(m/s)  UpperLimitTransitionRegionWidth=1e-4  UpperLimitTransitionRegionWidthUnits=m  TorqueActuationMode=ComputedTorque  MotionActuationMode=InputMotion  SensePosition=off  SenseVelocity=off  SenseAcceleration=off  SenseTorqueForce=off  SenseLowerLimitTorqueForce=off  SenseUpperLimitTorqueForce=off
  Joint3 : sm_lib/Joints/Revolute Joint  JointMode=Normal  CompositeWrenchDir=FollowerOnBase  CompositeWrenchFrame=BaseFrame  SenseConstraintForce=off  SenseConstraintTorque=off  SenseTotalForce=off  SenseTotalTorque=off  PositionTargetSpecify=off  PositionTargetPriority=High  PositionTargetValue=0  PositionTargetValueUnits=deg  VelocityTargetSpecify=off  VelocityTargetPriority=High  VelocityTargetValue=0  VelocityTargetValueUnits=deg/s  EquilibriumPosition=0  EquilibriumPositionUnits=deg  SpringStiffness=0  SpringStiffnessUnits=N*m/deg  DampingCoefficient=0  DampingCoefficientUnits=kg*m^2/(rad*s)  LowerLimitSpecify=on  LowerLimitBound=-3.14  LowerLimitBoundUnits=rad  LowerLimitStiffness=1e4  LowerLimitStiffnessUnits=N*m/deg  LowerLimitDamping=10  LowerLimitDampingUnits=N*m/(deg/s)  LowerLimitTransitionRegionWidth=0.1  LowerLimitTransitionRegionWidthUnits=deg  UpperLimitSpecify=on  UpperLimitBound=3.14  UpperLimitBoundUnits=rad  UpperLimitStiffness=1e4  UpperLimitStiffnessUnits=N*m/deg  UpperLimitDamping=10  UpperLimitDampingUnits=N*m/(deg/s)  UpperLimitTransitionRegionWidth=0.1  UpperLimitTransitionRegionWidthUnits=deg  TorqueActuationMode=ComputedTorque  MotionActuationMode=InputMotion  SensePosition=off  SenseVelocity=off  SenseAcceleration=off  SenseTorqueForce=off  SenseLowerLimitTorqueForce=off  SenseUpperLimitTorqueForce=off
  Link1 : Subsystem
  Link2 : Subsystem
  Link3 : Subsystem
  MechanismConfiguration : sm_lib/Utilities/Mechanism Configuration  UniformGravity=Constant  GravityVector=[0 0 -9.80665]  GravityVectorUnits=m/s^2  LinearizationDelta=0.001  JointModeTransitionNonlinearIterations=2
  Simulink-PS Converter1 : nesl_utility/Simulink-PS Converter  PhysicalDomain=network_engine_domain  SubClassName=ps_input  LeftPortType=input  RightPortType=output  PseudoPeriodic=off  Frequencies=[]  NoiseDistribution=none  NoiseParameters=[]  Unit=1  AffineConversion=off  FilteringAndDerivatives=filter  SimscapeFilterOrder=2  InputFilterTimeConstant=0.001  UdotUserProvided=0
  Simulink-PS Converter2 : nesl_utility/Simulink-PS Converter  PhysicalDomain=network_engine_domain  SubClassName=ps_input  LeftPortType=input  RightPortType=output  PseudoPeriodic=off  Frequencies=[]  NoiseDistribution=none  NoiseParameters=[]  Unit=1  AffineConversion=off  FilteringAndDerivatives=filter  SimscapeFilterOrder=2  InputFilterTimeConstant=0.001  UdotUserProvided=0
  Simulink-PS Converter3 : nesl_utility/Simulink-PS Converter  PhysicalDomain=network_engine_domain  SubClassName=ps_input  LeftPortType=input  RightPortType=output  PseudoPeriodic=off  Frequencies=[]  NoiseDistribution=none  NoiseParameters=[]  Unit=1  AffineConversion=off  FilteringAndDerivatives=filter  SimscapeFilterOrder=2  InputFilterTimeConstant=0.001  UdotUserProvided=0
  Solver Configuration : nesl_utility/Solver Configuration  PhysicalDomain=network_engine_domain  SubClassName=solver  LeftPortType=input  RightPortType=generic  Tones=[]  Harmonics=[]  SimulateNoise=off  Profile=off  UseLocalSampling=off  EnableSwitchedLinearOptims=on  FrequencyDomain=off  UseCCode=off  RelTol=0.001  AbsTol=0.001  MinStep=1e-09  ToWorkspace=off  RevertToSquareIcSolve=off  NumHomotopyIterations=100  PhasorMode=off  PhasorModeNumHarmonics=1  ConsistencySolver=NEWTON_XTOL_AFTER_FTOL  IndexReductionMethod=DerivativeReplacement  DoDC=off  ResidualTolerance=1e-09  ConsistencyTolSource=GLOBAL  ConsistencyAbsTol=0.001  ConsistencyRelTol=0.001  ConsistencyTolFactor=0.001  UseLocalSolver=off  LocalSolverChoice=NE_BACKWARD_EULER_ADVANCER  ResolveIndetEquations=on  FunctionEvalNumThread=1  LocalSolverSampleTime=0.001  DoFixedCost=off  MaxNonlinIter=3  MaxModeIter=2  ComputeImpulses=off  ImpulseIterations=2  LinearAlgebra=auto  LinearAlgebraNumThread=0  EquationFormulation=NE_TIME_EF  DelaysMemoryBudget=1024  AutomaticFiltering=on  FilteringTimeConstant=0.001  PartitionStorageMethod=AS_NEEDED  PartitionMemoryBudget=1024  PartitionMethod=ROBUST  MultibodyUseLocalSolver=off  MultibodyLocalSolverChoice=ODE1  MultibodyLocalSolverSampleTime=0.001
  Visual : sm_lib/Body Elements/Cylindrical Solid  CylinderRadius=0.02  CylinderRadiusUnits=m  CylinderLength=0.01  CylinderLengthUnits=m  ExportEntireGeometry=off  InertiaType=Custom  BasedOnType=Density  Density=1000  DensityUnits=kg/m^3  Mass=0  MassUnits=kg  CenterOfMass=[0, 0, 0]  CenterOfMassUnits=m  MomentsOfInertia=[0, 0, 0]  MomentsOfInertiaUnits=kg*m^2  ProductsOfInertia=[0, 0, 0]  ProductsOfInertiaUnits=kg*m^2  GraphicType=FromGeometry  MarkerShape=Sphere  MarkerSize=10  GraphicVisPropType=SimpleVisualProperties  GraphicDiffuseColor=[1, 1, 0]  GraphicOpacity=1  GraphicSpecularColor=[0.5 0.5 0.5 1.0]  GraphicAmbientColor=[0.15 0.15 0.15 1.0]  GraphicEmissiveColor=[0.0 0.0 0.0 1.0]  GraphicShininess=75  DoExposeReferenceFrame=on  SerializedFrames=<Frames/>
  Visual1 : sm_lib/Body Elements/Brick Solid  BrickDimensions=[0.4, 0.4, 0.1]  BrickDimensionsUnits=m  ExportEntireGeometry=off  InertiaType=Custom  BasedOnType=Density  Density=1000  DensityUnits=kg/m^3  Mass=0  MassUnits=kg  CenterOfMass=[0, 0, 0]  CenterOfMassUnits=m  MomentsOfInertia=[0, 0, 0]  MomentsOfInertiaUnits=kg*m^2  ProductsOfInertia=[0, 0, 0]  ProductsOfInertiaUnits=kg*m^2  GraphicType=FromGeometry  MarkerShape=Sphere  MarkerSize=10  GraphicVisPropType=SimpleVisualProperties  GraphicDiffuseColor=[1 0.4118 0.1608]  GraphicOpacity=0.6  GraphicSpecularColor=[0.5 0.5 0.5 1.0]  GraphicAmbientColor=[0.15 0.15 0.15 1.0]  GraphicEmissiveColor=[0.0 0.0 0.0 1.0]  GraphicShininess=75  DoExposeReferenceFrame=on  SerializedFrames=<Frames/>
  VisualOrigin1Transform : sm_lib/Frames and Transforms/Rigid Transform  RotationMethod=RotationSequence  FollAlignAxisA=+X  BaseAlignAxisA=+Y  FollAlignAxisB=+Y  BaseAlignAxisB=+Z  RotationStandardAxis=+Z  RotationAngle=0  RotationAngleUnits=deg  RotationArbitraryAxis=[0 0 1]  RotationSequenceAxes=BaseAxes  RotationSequence=XYZ  RotationSequenceAngles=[pi/2, 0, 0]  RotationSequenceAnglesUnits=rad  RotationMatrix=[1 0 0;0 1 0;0 0 1]  Quaternion=[1 0 0 0]  TranslationMethod=Cartesian  TranslationCartesianOffset=[0.4, -0.45, 0.2]  TranslationCartesianOffsetUnits=m  TranslationStandardAxis=+Z  TranslationStandardOffset=0  TranslationStandardOffsetUnits=m  TranslationROffset=0  TranslationROffsetUnits=m  TranslationThetaOffset=0  TranslationThetaOffsetUnits=deg  TranslationZOffset=0  TranslationZOffsetUnits=m
  VisualOrigin1Transform1 : sm_lib/Frames and Transforms/Rigid Transform  RotationMethod=RotationSequence  FollAlignAxisA=+X  BaseAlignAxisA=+Y  FollAlignAxisB=+Y  BaseAlignAxisB=+Z  RotationStandardAxis=+Z  RotationAngle=0  RotationAngleUnits=deg  RotationArbitraryAxis=[0 0 1]  RotationSequenceAxes=BaseAxes  RotationSequence=XYZ  RotationSequenceAngles=[0, 0, 0]  RotationSequenceAnglesUnits=rad  RotationMatrix=[1 0 0;0 1 0;0 0 1]  Quaternion=[1 0 0 0]  TranslationMethod=Cartesian  TranslationCartesianOffset=[0.4 -0.54 0.15]  TranslationCartesianOffsetUnits=m  TranslationStandardAxis=+Z  TranslationStandardOffset=0  TranslationStandardOffsetUnits=m  TranslationROffset=0  TranslationROffsetUnits=m  TranslationThetaOffset=0  TranslationThetaOffsetUnits=deg  TranslationZOffset=0  TranslationZOffsetUnits=m
  World : sm_lib/Frames and Transforms/World Frame
  base_link : Subsystem
  ee : Subsystem
  ee_link : sm_lib/Joints/Weld Joint  JointMode=Normal  CompositeWrenchDir=FollowerOnBase  CompositeWrenchFrame=BaseFrame  SenseConstraintForce=off  SenseConstraintTorque=off  SenseTotalForce=off  SenseTotalTorque=off
  wires:
  In3/1 -> Simulink-PS Converter2/1
  In1/1 -> Simulink-PS Converter3/1
  In2/1 -> Simulink-PS Converter1/1
  connections:
  Simulink-PS Converter3/RConn1 -- Joint1/LConn2
  Simulink-PS Converter1/RConn1 -- Joint2/LConn2
  Joint3/LConn2 -- Simulink-PS Converter2/RConn1
  World/RConn1 -- VisualOrigin1Transform1/LConn1 -- VisualOrigin1Transform/LConn1 -- base_link/LConn1 -- MechanismConfiguration/RConn1 -- Solver Configuration/RConn1
  Joint2/RConn1 -- Link2/LConn1
  Joint2/LConn1 -- Link1/RConn1
  Joint3/LConn1 -- Link2/RConn1
  Link3/RConn1 -- ee_link/LConn1
  ee/LConn1 -- ee_link/RConn1
  Joint1/RConn1 -- Link1/LConn1
  Joint3/RConn1 -- Link3/LConn1
  Joint1/LConn1 -- base_link/RConn1
  VisualOrigin1Transform/RConn1 -- Visual1/RConn1
  VisualOrigin1Transform1/RConn1 -- Visual/RConn1

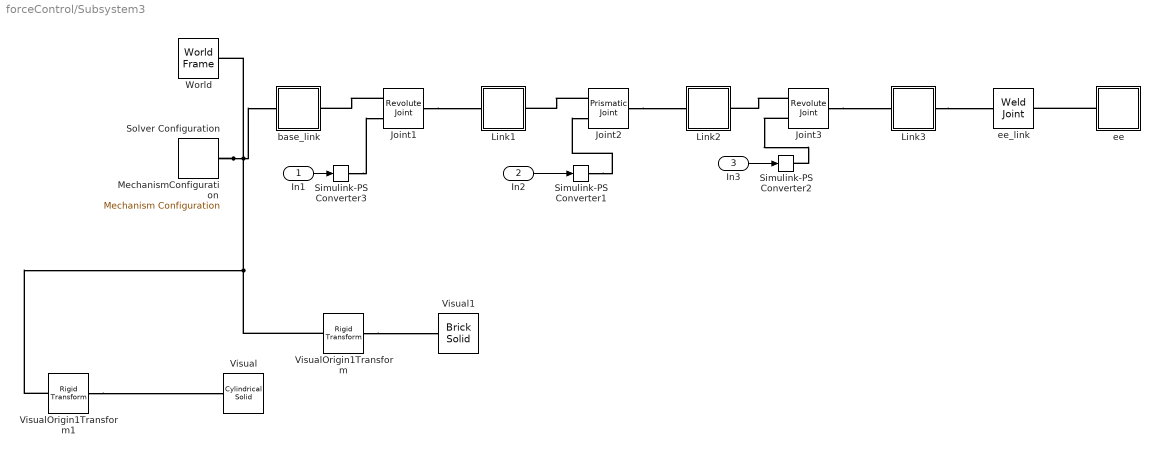
== system forceControl/Subsystem3 ==
  In1 : Inport
  In2 : Inport  Port=2
  In3 : Inport  Port=3
  Joint1 : sm_lib/Joints/Revolute Joint  JointMode=Normal  CompositeWrenchDir=FollowerOnBase  CompositeWrenchFrame=BaseFrame  SenseConstraintForce=off  SenseConstraintTorque=off  SenseTotalForce=off  SenseTotalTorque=off  PositionTargetSpecify=off  PositionTargetPriority=High  PositionTargetValue=0  PositionTargetValueUnits=deg  VelocityTargetSpecify=off  VelocityTargetPriority=High  VelocityTargetValue=0  VelocityTargetValueUnits=deg/s  EquilibriumPosition=0  EquilibriumPositionUnits=deg  SpringStiffness=0  SpringStiffnessUnits=N*m/deg  DampingCoefficient=0  DampingCoefficientUnits=kg*m^2/(rad*s)  LowerLimitSpecify=on  LowerLimitBound=-3.14  LowerLimitBoundUnits=rad  LowerLimitStiffness=1e4  LowerLimitStiffnessUnits=N*m/deg  LowerLimitDamping=10  LowerLimitDampingUnits=N*m/(deg/s)  LowerLimitTransitionRegionWidth=0.1  LowerLimitTransitionRegionWidthUnits=deg  UpperLimitSpecify=on  UpperLimitBound=3.14  UpperLimitBoundUnits=rad  UpperLimitStiffness=1e4  UpperLimitStiffnessUnits=N*m/deg  UpperLimitDamping=10  UpperLimitDampingUnits=N*m/(deg/s)  UpperLimitTransitionRegionWidth=0.1  UpperLimitTransitionRegionWidthUnits=deg  TorqueActuationMode=ComputedTorque  MotionActuationMode=InputMotion  SensePosition=off  SenseVelocity=off  SenseAcceleration=off  SenseTorqueForce=off  SenseLowerLimitTorqueForce=off  SenseUpperLimitTorqueForce=off
  Joint2 : sm_lib/Joints/Prismatic Joint  JointMode=Normal  CompositeWrenchDir=FollowerOnBase  CompositeWrenchFrame=BaseFrame  SenseConstraintForce=off  SenseConstraintTorque=off  SenseTotalForce=off  SenseTotalTorque=off  PositionTargetSpecify=off  PositionTargetPriority=High  PositionTargetValue=0  PositionTargetValueUnits=m  VelocityTargetSpecify=off  VelocityTargetPriority=High  VelocityTargetValue=0  VelocityTargetValueUnits=m/s  EquilibriumPosition=0  EquilibriumPositionUnits=m  SpringStiffness=0  SpringStiffnessUnits=N/m  DampingCoefficient=0  DampingCoefficientUnits=kg/s  LowerLimitSpecify=on  LowerLimitBound=-0.3  LowerLimitBoundUnits=m  LowerLimitStiffness=1e6  LowerLimitStiffnessUnits=N/m  LowerLimitDamping=1e3  LowerLimitDampingUnits=N/(m/s)  LowerLimitTransitionRegionWidth=1e-4  LowerLimitTransitionRegionWidthUnits=m  UpperLimitSpecify=on  UpperLimitBound=0  UpperLimitBoundUnits=m  UpperLimitStiffness=1e6  UpperLimitStiffnessUnits=N/m  UpperLimitDamping=1e3  UpperLimitDampingUnits=N/(m/s)  UpperLimitTransitionRegionWidth=1e-4  UpperLimitTransitionRegionWidthUnits=m  TorqueActuationMode=ComputedTorque  MotionActuationMode=InputMotion  SensePosition=off  SenseVelocity=off  SenseAcceleration=off  SenseTorqueForce=off  SenseLowerLimitTorqueForce=off  SenseUpperLimitTorqueForce=off
  Joint3 : sm_lib/Joints/Revolute Joint  JointMode=Normal  CompositeWrenchDir=FollowerOnBase  CompositeWrenchFrame=BaseFrame  SenseConstraintForce=off  SenseConstraintTorque=off  SenseTotalForce=off  SenseTotalTorque=off  PositionTargetSpecify=off  PositionTargetPriority=High  PositionTargetValue=0  PositionTargetValueUnits=deg  VelocityTargetSpecify=off  VelocityTargetPriority=High  VelocityTargetValue=0  VelocityTargetValueUnits=deg/s  EquilibriumPosition=0  EquilibriumPositionUnits=deg  SpringStiffness=0  SpringStiffnessUnits=N*m/deg  DampingCoefficient=0  DampingCoefficientUnits=kg*m^2/(rad*s)  LowerLimitSpecify=on  LowerLimitBound=-3.14  LowerLimitBoundUnits=rad  LowerLimitStiffness=1e4  LowerLimitStiffnessUnits=N*m/deg  LowerLimitDamping=10  LowerLimitDampingUnits=N*m/(deg/s)  LowerLimitTransitionRegionWidth=0.1  LowerLimitTransitionRegionWidthUnits=deg  UpperLimitSpecify=on  UpperLimitBound=3.14  UpperLimitBoundUnits=rad  UpperLimitStiffness=1e4  UpperLimitStiffnessUnits=N*m/deg  UpperLimitDamping=10  UpperLimitDampingUnits=N*m/(deg/s)  UpperLimitTransitionRegionWidth=0.1  UpperLimitTransitionRegionWidthUnits=deg  TorqueActuationMode=ComputedTorque  MotionActuationMode=InputMotion  SensePosition=off  SenseVelocity=off  SenseAcceleration=off  SenseTorqueForce=off  SenseLowerLimitTorqueForce=off  SenseUpperLimitTorqueForce=off
  Link1 : Subsystem
  Link2 : Subsystem
  Link3 : Subsystem
  MechanismConfiguration : sm_lib/Utilities/Mechanism Configuration  UniformGravity=Constant  GravityVector=[0 0 -9.80665]  GravityVectorUnits=m/s^2  LinearizationDelta=0.001  JointModeTransitionNonlinearIterations=2
  Simulink-PS Converter1 : nesl_utility/Simulink-PS Converter  PhysicalDomain=network_engine_domain  SubClassName=ps_input  LeftPortType=input  RightPortType=output  PseudoPeriodic=off  Frequencies=[]  NoiseDistribution=none  NoiseParameters=[]  Unit=1  AffineConversion=off  FilteringAndDerivatives=filter  SimscapeFilterOrder=2  InputFilterTimeConstant=0.001  UdotUserProvided=0
  Simulink-PS Converter2 : nesl_utility/Simulink-PS Converter  PhysicalDomain=network_engine_domain  SubClassName=ps_input  LeftPortType=input  RightPortType=output  PseudoPeriodic=off  Frequencies=[]  NoiseDistribution=none  NoiseParameters=[]  Unit=1  AffineConversion=off  FilteringAndDerivatives=filter  SimscapeFilterOrder=2  InputFilterTimeConstant=0.001  UdotUserProvided=0
  Simulink-PS Converter3 : nesl_utility/Simulink-PS Converter  PhysicalDomain=network_engine_domain  SubClassName=ps_input  LeftPortType=input  RightPortType=output  PseudoPeriodic=off  Frequencies=[]  NoiseDistribution=none  NoiseParameters=[]  Unit=1  AffineConversion=off  FilteringAndDerivatives=filter  SimscapeFilterOrder=2  InputFilterTimeConstant=0.001  UdotUserProvided=0
  Solver Configuration : nesl_utility/Solver Configuration  PhysicalDomain=network_engine_domain  SubClassName=solver  LeftPortType=input  RightPortType=generic  Tones=[]  Harmonics=[]  SimulateNoise=off  Profile=off  UseLocalSampling=off  EnableSwitchedLinearOptims=on  FrequencyDomain=off  UseCCode=off  RelTol=0.001  AbsTol=0.001  MinStep=1e-09  ToWorkspace=off  RevertToSquareIcSolve=off  NumHomotopyIterations=100  PhasorMode=off  PhasorModeNumHarmonics=1  ConsistencySolver=NEWTON_XTOL_AFTER_FTOL  IndexReductionMethod=DerivativeReplacement  DoDC=off  ResidualTolerance=1e-09  ConsistencyTolSource=GLOBAL  ConsistencyAbsTol=0.001  ConsistencyRelTol=0.001  ConsistencyTolFactor=0.001  UseLocalSolver=off  LocalSolverChoice=NE_BACKWARD_EULER_ADVANCER  ResolveIndetEquations=on  FunctionEvalNumThread=1  LocalSolverSampleTime=0.001  DoFixedCost=off  MaxNonlinIter=3  MaxModeIter=2  ComputeImpulses=off  ImpulseIterations=2  LinearAlgebra=auto  LinearAlgebraNumThread=0  EquationFormulation=NE_TIME_EF  DelaysMemoryBudget=1024  AutomaticFiltering=on  FilteringTimeConstant=0.001  PartitionStorageMethod=AS_NEEDED  PartitionMemoryBudget=1024  PartitionMethod=ROBUST  MultibodyUseLocalSolver=off  MultibodyLocalSolverChoice=ODE1  MultibodyLocalSolverSampleTime=0.001
  Visual : sm_lib/Body Elements/Cylindrical Solid  CylinderRadius=0.02  CylinderRadiusUnits=m  CylinderLength=0.01  CylinderLengthUnits=m  ExportEntireGeometry=off  InertiaType=Custom  BasedOnType=Density  Density=1000  DensityUnits=kg/m^3  Mass=0  MassUnits=kg  CenterOfMass=[0, 0, 0]  CenterOfMassUnits=m  MomentsOfInertia=[0, 0, 0]  MomentsOfInertiaUnits=kg*m^2  ProductsOfInertia=[0, 0, 0]  ProductsOfInertiaUnits=kg*m^2  GraphicType=FromGeometry  MarkerShape=Sphere  MarkerSize=10  GraphicVisPropType=SimpleVisualProperties  GraphicDiffuseColor=[1, 1, 0]  GraphicOpacity=1  GraphicSpecularColor=[0.5 0.5 0.5 1.0]  GraphicAmbientColor=[0.15 0.15 0.15 1.0]  GraphicEmissiveColor=[0.0 0.0 0.0 1.0]  GraphicShininess=75  DoExposeReferenceFrame=on  SerializedFrames=<Frames/>
  Visual1 : sm_lib/Body Elements/Brick Solid  BrickDimensions=[0.4, 0.4, 0.1]  BrickDimensionsUnits=m  ExportEntireGeometry=off  InertiaType=Custom  BasedOnType=Density  Density=1000  DensityUnits=kg/m^3  Mass=0  MassUnits=kg  CenterOfMass=[0, 0, 0]  CenterOfMassUnits=m  MomentsOfInertia=[0, 0, 0]  MomentsOfInertiaUnits=kg*m^2  ProductsOfInertia=[0, 0, 0]  ProductsOfInertiaUnits=kg*m^2  GraphicType=FromGeometry  MarkerShape=Sphere  MarkerSize=10  GraphicVisPropType=SimpleVisualProperties  GraphicDiffuseColor=[1 0.4118 0.1608]  GraphicOpacity=0.6  GraphicSpecularColor=[0.5 0.5 0.5 1.0]  GraphicAmbientColor=[0.15 0.15 0.15 1.0]  GraphicEmissiveColor=[0.0 0.0 0.0 1.0]  GraphicShininess=75  DoExposeReferenceFrame=on  SerializedFrames=<Frames/>
  VisualOrigin1Transform : sm_lib/Frames and Transforms/Rigid Transform  RotationMethod=RotationSequence  FollAlignAxisA=+X  BaseAlignAxisA=+Y  FollAlignAxisB=+Y  BaseAlignAxisB=+Z  RotationStandardAxis=+Z  RotationAngle=0  RotationAngleUnits=deg  RotationArbitraryAxis=[0 0 1]  RotationSequenceAxes=BaseAxes  RotationSequence=XYZ  RotationSequenceAngles=[pi/2, 0, 0]  RotationSequenceAnglesUnits=rad  RotationMatrix=[1 0 0;0 1 0;0 0 1]  Quaternion=[1 0 0 0]  TranslationMethod=Cartesian  TranslationCartesianOffset=[0.4, -0.45, 0.2]  TranslationCartesianOffsetUnits=m  TranslationStandardAxis=+Z  TranslationStandardOffset=0  TranslationStandardOffsetUnits=m  TranslationROffset=0  TranslationROffsetUnits=m  TranslationThetaOffset=0  TranslationThetaOffsetUnits=deg  TranslationZOffset=0  TranslationZOffsetUnits=m
  VisualOrigin1Transform1 : sm_lib/Frames and Transforms/Rigid Transform  RotationMethod=RotationSequence  FollAlignAxisA=+X  BaseAlignAxisA=+Y  FollAlignAxisB=+Y  BaseAlignAxisB=+Z  RotationStandardAxis=+Z  RotationAngle=0  RotationAngleUnits=deg  RotationArbitraryAxis=[0 0 1]  RotationSequenceAxes=BaseAxes  RotationSequence=XYZ  RotationSequenceAngles=[0, 0, 0]  RotationSequenceAnglesUnits=rad  RotationMatrix=[1 0 0;0 1 0;0 0 1]  Quaternion=[1 0 0 0]  TranslationMethod=Cartesian  TranslationCartesianOffset=[0.4 -0.54 0.15]  TranslationCartesianOffsetUnits=m  TranslationStandardAxis=+Z  TranslationStandardOffset=0  TranslationStandardOffsetUnits=m  TranslationROffset=0  TranslationROffsetUnits=m  TranslationThetaOffset=0  TranslationThetaOffsetUnits=deg  TranslationZOffset=0  TranslationZOffsetUnits=m
  World : sm_lib/Frames and Transforms/World Frame
  base_link : Subsystem
  ee : Subsystem
  ee_link : sm_lib/Joints/Weld Joint  JointMode=Normal  CompositeWrenchDir=FollowerOnBase  CompositeWrenchFrame=BaseFrame  SenseConstraintForce=off  SenseConstraintTorque=off  SenseTotalForce=off  SenseTotalTorque=off
  wires:
  In3/1 -> Simulink-PS Converter2/1
  In1/1 -> Simulink-PS Converter3/1
  In2/1 -> Simulink-PS Converter1/1
  connections:
  Simulink-PS Converter3/RConn1 -- Joint1/LConn2
  Simulink-PS Converter1/RConn1 -- Joint2/LConn2
  Joint3/LConn2 -- Simulink-PS Converter2/RConn1
  World/RConn1 -- VisualOrigin1Transform1/LConn1 -- VisualOrigin1Transform/LConn1 -- base_link/LConn1 -- MechanismConfiguration/RConn1 -- Solver Configuration/RConn1
  Joint2/RConn1 -- Link2/LConn1
  Joint2/LConn1 -- Link1/RConn1
  Joint3/LConn1 -- Link2/RConn1
  Link3/RConn1 -- ee_link/LConn1
  ee/LConn1 -- ee_link/RConn1
  Joint1/RConn1 -- Link1/LConn1
  Joint3/RConn1 -- Link3/LConn1
  Joint1/LConn1 -- base_link/RConn1
  VisualOrigin1Transform/RConn1 -- Visual1/RConn1
  VisualOrigin1Transform1/RConn1 -- Visual/RConn1
